simulink model "Circuit"  (R2020b)
settings: Solver=VariableStepAuto  StartTime=0.0  StopTime=10.0  RelTol=1e-3
undefined symbols (not defined in the file): C, R
settings Model: Creator=Shubham  LastModifiedBy=Shubham
settings DataIOCC: ExternalInput=[t, E]  LoadExternalInput=on  SaveFormat=Array

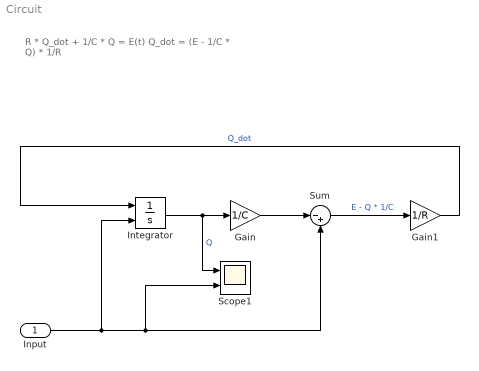
== system Circuit ==
  note: R * Q_dot + 1/C * Q = E(t)
      |
      | Q_dot = (E - 1/C * Q) * 1/R
  Input : Inport
  Gain : Gain  Gain=1/C
  Gain1 : Gain  Gain=1/R
  Integrator : Integrator  InitialConditionSource=external  InitialCondition=4
  Scope1 : Scope  NumInputPorts=2
  Sum : Sum  Inputs=|-+
  wires:
  Gain1/1 -> Integrator/1  "Q_dot"
  Integrator/1 -> Scope1/1, Gain/1  "Q"
  Gain/1 -> Sum/1
  Sum/1 -> Gain1/1  "E - Q * 1/C"
  Input/1 -> Integrator/2, Scope1/2, Sum/2
